simulink model "SoftStart"  (R2021a)
settings: Solver=ode45  StartTime=0.0  StopTime=10  RelTol=1e-3  EnableMultiTasking=on
undefined symbols (not defined in the file or in its folder): D1, lagging, pulse
libraries: spsThyristorLib x6, spsACVoltageSourceLib x3, spsAsynchronousMachineSIUnitsLib x2, spsThreePhaseVIMeasurementLib x2, spsPulseGeneratorThyristor12PulseLib x1, spsGroundLib x1, spsPLL3phLib x1, spspowerguiLib x1
settings Model: Creator=khaled18  LastModifiedBy=dudekpob
settings SolverCC: AlgebraicLoopSolver=TrustRegion
settings DataIOCC: LimitDataPoints=on  SaveFormat=Array  ReturnWorkspaceOutputs=off
settings OptimizationCC: LifeSpan=inf
settings DebuggingCC: SolverPrmCheckMsg=warning  SFUnexpectedBacktrackingDiag=warning  SFNoUnconditionalDefaultTransitionDiag=warning  SFExecutionAtInitializationDiag=none  SFMachineParentedDataDiag=warning  ArithmeticOperatorsInVariantConditions=warning
settings HardwareCC: ProdBitPerPointer=32  ProdBitPerSizeT=32  ProdBitPerPtrDiffT=32  ProdLargestAtomicFloat=None  ProdIntDivRoundTo=Undefined  ProdEndianess=Unspecified  ProdWordSize=32  ProdHWDeviceType=32-bit Generic
settings ModelReferenceCC: PropagateSignalLabelsOutOfModel=off
settings SFSimCC: SimUseLocalCustomCode=off  CustomCodeUndefinedFunction=UseInterfaceOnly
settings RTWCC: RTWUseLocalCustomCode=off
settings CodeAppCC: StateflowObjectComments=on
settings GRTTargetCC: TargetLangStandard=C89/C90 (ANSI)
settings ConfigComp: CovMetricSettings=dw  CovSaveCumulativeToWorkspaceVar=on  CovSaveSingleToWorkspaceVar=on  CovExternalEMLEnable=off  CovSFcnEnable=off
settings SimscapeCC: SimscapeNormalizeSystem=off

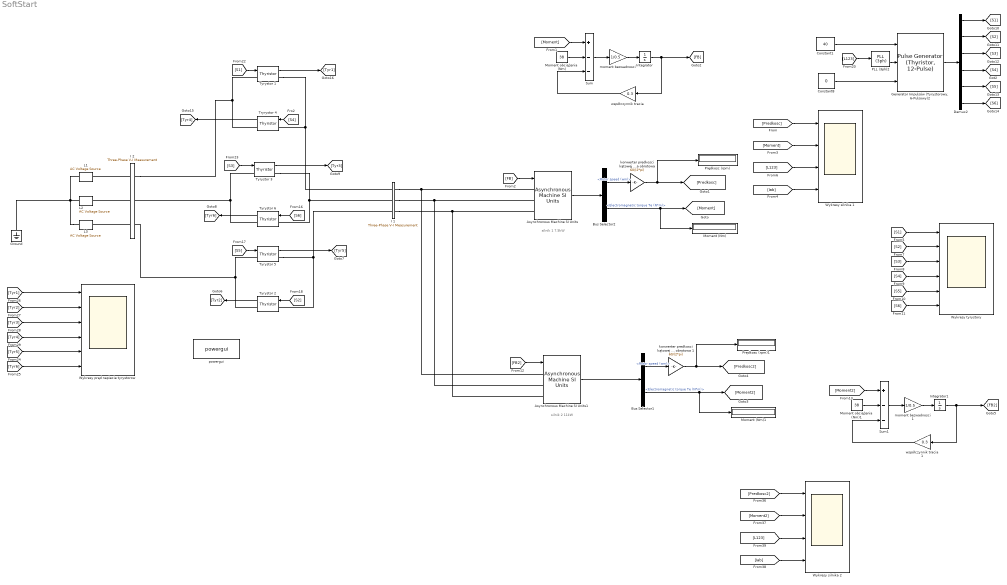
== system SoftStart ==
  note: silnik 1 7.5kW
  note: silnik 2 11kW
  Asynchronous Machine SI Units : spsAsynchronousMachineSIUnitsLib/Asynchronous Machine SI Units  RotorType=Squirrel-cage  PresetModel=No  MechanicalLoad=Speed w  ShowDetailedParameters=on  ReferenceFrame=Rotor  Units=SI  MeasurementBus=off  NominalParameters=[7500 400 50]  VoltageRatio=1  Stator=[1.405 0.005839]  Rotor=[1.395 0.005839]  Cage1=[ 0.022 0.226/377]  Cage2=[ 0.022 0.226/377]  Lm=0.1722  Mechanical=[0.0131 0.002985 3]  PolePairs=3  InitialConditions=[1 0 0 0 0 0 0 0]  SimulateSaturation=on  Saturation=[14.03593122, 27.81365428, 53.79336849, 72.68890987, 97.98006896, 148.6815601, 215.7428561, 302.9841135, 428.7778367 ; 230, 322, 414, 460, 506, 552, 598, 644, 690]  LoadFlowParameters=1492000  TsPowergui=0  TsBlock=-1  IterativeModel=Forward Euler  IterativeDiscreteModel=Trapezoidal non iterative  Pmec=0
      settings: AttributesFormatString=\n
  Asynchronous Machine SI Units1 : spsAsynchronousMachineSIUnitsLib/Asynchronous Machine SI Units  RotorType=Squirrel-cage  PresetModel=No  MechanicalLoad=Speed w  ShowDetailedParameters=on  ReferenceFrame=Rotor  Units=SI  MeasurementBus=off  NominalParameters=[11000 400 50]  VoltageRatio=1  Stator=[1.405 0.005839]  Rotor=[1.395 0.005839]  Cage1=[ 0.022 0.226/377]  Cage2=[ 0.022 0.226/377]  Lm=0.1722  Mechanical=[0.0131 0.002985 3]  PolePairs=3  InitialConditions=[1 0 0 0 0 0 0 0]  SimulateSaturation=on  Saturation=[14.03593122, 27.81365428, 53.79336849, 65.68890987, 75.98006896, 85.6815601, 90.7428561, 100.9841135, 110.7778367 ; 230, 322, 414, 460, 506, 552, 598, 644, 690]  LoadFlowParameters=1492000  TsPowergui=0  TsBlock=-1  IterativeModel=Forward Euler  IterativeDiscreteModel=Trapezoidal non iterative  Pmec=0
      settings: AttributesFormatString=\n
  Bus Selector1 : BusSelector  OutputSignals=Mechanical.Rotor speed (wm),Mechanical.Electromagnetic torque Te (N*m)
  Bus Selector2 : BusSelector  OutputSignals=Mechanical.Rotor speed (wm),Mechanical.Electromagnetic torque Te (N*m)
  Constant1 : Constant  Value=40
  Constant8 : Constant  Value=0
  Demux2 : Demux  Outputs=6
  "Generator Impulsów (Tyrystorowy, 6-Pulsowy)2" : spsPulseGeneratorThyristor12PulseLib/Pulse Generator (Thyristor, 12-Pulse)  GenType=6-pulse  Delta=D1 (lagging)  pwidth=50  Double_Pulse=on  Ts=0
      settings: SourceProductBaseCode=PS
  Ground : spsGroundLib/Ground  LConnTagsString=a
  I 1 : spsThreePhaseVIMeasurementLib/Three-Phase V-I Measurement  VoltageMeasurement=phase-to-phase  SetLabelV=on  LabelV=Vabc1  Vpu=off  VpuLL=off  CurrentMeasurement=yes  SetLabelI=on  LabelI=Iabc1  Ipu=off  Pbase=100e6  Vbase=500e3  OutputType=Complex  PhasorSimulation=off  PSBequivalent=0
  I 2 : spsThreePhaseVIMeasurementLib/Three-Phase V-I Measurement  VoltageMeasurement=phase-to-ground  SetLabelV=on  LabelV=L123  Vpu=off  VpuLL=off  CurrentMeasurement=yes  SetLabelI=on  LabelI=Iab  Ipu=off  Pbase=100e6  Vbase=500e3  OutputType=Complex  PhasorSimulation=off  PSBequivalent=0
  Integrator : Integrator
  Integrator1 : Integrator
  L1 : spsACVoltageSourceLib/AC Voltage Source  Amplitude=400  Phase=0  Frequency=50  SampleTime=0  Measurements=None  BusType=swing  Pref=10e3  Qref=0  Qmin=-inf  Qmax=+inf
  L2 : spsACVoltageSourceLib/AC Voltage Source  Amplitude=400  Phase=-120  Frequency=50  SampleTime=0  Measurements=None  BusType=swing  Pref=10e3  Qref=0  Qmin=-inf  Qmax=+inf
  L3 : spsACVoltageSourceLib/AC Voltage Source  Amplitude=400  Phase=120  Frequency=50  SampleTime=0  Measurements=None  BusType=swing  Pref=10e3  Qref=0  Qmin=-inf  Qmax=+inf
  Moment (Nm) : Display
  Moment (Nm)1 : Display
  Moment obciążenia  (Nm) : Constant  Value=38
  Moment obciążenia  (Nm)1 : Constant  Value=38
  PLL (3ph)2 : spsPLL3phLib/PLL (3ph)  Fmin=45  Par_Init=[0, 50]  ParK=[180, 3200, 1]  TcD=1e-4  MaxRateChangeFreq=12  FilterCutOffFreq=25  Ts=0  AGC=on
  Prędkosc (rpm) : Display
  Prędkosc (rpm)1 : Display
  Sum : Sum  Inputs=+--
  Sum1 : Sum  Inputs=+--
  Tryrystor 4 : spsThyristorLib/Thyristor  Ron=0.001  Lon=0  Vf=0.8  IC=0  Rs=500  Cs=250e-9  Measurements=on
  Tyrystor {1..3,5..6} (5 alike) : spsThyristorLib/Thyristor  Ron=0.001  Lon=0  Vf=0.8  IC=0  Rs=500  Cs=250e-9  Measurements=on
  Wykresy prąd napiecie tyrystorow : Scope  NumInputPorts=6
  Wykresy silnika 1 : Scope  NumInputPorts=4
  Wykresy silnika 2 : Scope  NumInputPorts=4
  Wykresy tyrystory : Scope  NumInputPorts=6
  "konwerter predkosci kątowej na obrotowa " : Gain  Gain=60/(2*pi)
  konwerter predkosci kątowej na obrotowa 1 : Gain  Gain=60/(2*pi)
  moment bezwadnosci : Gain  Gain=1/0.5
  moment bezwadnosci1 : Gain  Gain=1/0.5
  powergui : spspowerguiLib/powergui  Priority=1  SimulationMode=Discrete  SampleTime=50e-6  frequency=60  Iterations=50  frequencyindice=50  Pbase=100e6  ErrMax=1e-4  UnitsV=kV  UnitsW=MW  buscounter=0  FunctionMessages=off  echomessages=off  EnableUseOfTLC=off  CurrentSourceSwitches=off  DisableSnubberDevices=off  DisableRonSwitches=off  DisableVfSwitches=off  DisplayEquations=off  AutomaticDiscreteSolvers=off  SolverType=Tustin/Backward Euler (TBE)  Interpol=off  ExternalGateDelay=off  methode=off  Ts=100  x0status=blocks  SPID=off  SwTol=0  HookPort=off  NonlinearTolerance=1e-4  nMaxIteration=100  ContinueOnMaxIteration=off  RestoreLinks=warning  ResistiveCurrentMeasurement=off  Frange=[0:2:500]  Ylog=off  Xlog=on  ShowGrid=off  save=off  variable=ZData  structure=0  ZoomFFT=off  StartTime=0.0  cycles=1  DisplayStyle=1  fundamental=60  FreqAxis=off  MaxFrequency=1000  frequencyindicesteady=1  RmsSteady=1  display=off
  "współczynnik tracia " : Gain  Gain=0.3
  współczynnik tracia 1 : Gain  Gain=0.3
  wires:
  [L123] -> PLL (3ph)2/1
  Constant8/1 -> "Generator Impulsów (Tyrystorowy, 6-Pulsowy)2"/3
  "Generator Impulsów (Tyrystorowy, 6-Pulsowy)2"/1 -> Demux2/1
  [S4] -> Tryrystor 4/1
  [S5] -> Tyrystor 5/1
  Demux2/4 -> [S4]
  Asynchronous Machine SI Units/1 -> Bus Selector2/1
  [S6] -> Tyrystor 6/1
  Demux2/5 -> [S5]
  Demux2/2 -> [S2]
  Demux2/6 -> [S6]
  PLL (3ph)2/2 -> "Generator Impulsów (Tyrystorowy, 6-Pulsowy)2"/2
  [S1] -> Tyrystor 1/1
  Demux2/1 -> [S1]
  [S3] -> Tyrystor 3/1
  Demux2/3 -> [S3]
  [S2] -> Tyrystor 2/1
  Constant1/1 -> "Generator Impulsów (Tyrystorowy, 6-Pulsowy)2"/1
  Bus Selector2/2 -> Moment (Nm)/1, [Moment]  "<Electromagnetic torque Te (N*m)>"
  Sum/1 -> moment bezwadnosci/1
  moment bezwadnosci/1 -> Integrator/1
  Integrator/1 -> "współczynnik tracia "/1, [FB]
  Bus Selector2/1 -> "konwerter predkosci kątowej na obrotowa "/1  "<Rotor speed (wm)>"
  [Moment] -> Sum/1
  Moment obciążenia  (Nm)/1 -> Sum/2
  "współczynnik tracia "/1 -> Sum/3
  [FB] -> Asynchronous Machine SI Units/1
  "konwerter predkosci kątowej na obrotowa "/1 -> Prędkosc (rpm)/1, [Predkosc]
  [Predkosc] -> Wykresy silnika 1/1
  [Moment] -> Wykresy silnika 1/2
  [L123] -> Wykresy silnika 1/3
  [Iab] -> Wykresy silnika 1/4
  [S1] -> Wykresy tyrystory/1
  [S2] -> Wykresy tyrystory/2
  [S3] -> Wykresy tyrystory/3
  [S4] -> Wykresy tyrystory/4
  [S5] -> Wykresy tyrystory/5
  [S6] -> Wykresy tyrystory/6
  [Tyr4] -> Wykresy prąd napiecie tyrystorow/4
  [Tyr1] -> Wykresy prąd napiecie tyrystorow/1
  [Tyr3] -> Wykresy prąd napiecie tyrystorow/3
  [Tyr2] -> Wykresy prąd napiecie tyrystorow/2
  [Tyr6] -> Wykresy prąd napiecie tyrystorow/6
  [Tyr5] -> Wykresy prąd napiecie tyrystorow/5
  Tyrystor 2/1 -> [Tyr2]
  Tyrystor 5/1 -> [Tyr5]
  Tyrystor 6/1 -> [Tyr6]
  Tyrystor 3/1 -> [Tyr3]
  Tryrystor 4/1 -> [Tyr4]
  Tyrystor 1/1 -> [Tyr1]
  [Predkosc2] -> Wykresy silnika 2/1
  [Iab] -> Wykresy silnika 2/4
  [Moment2] -> Wykresy silnika 2/2
  [L123] -> Wykresy silnika 2/3
  [FB2] -> Asynchronous Machine SI Units1/1
  Bus Selector1/1 -> konwerter predkosci kątowej na obrotowa 1/1  "<Rotor speed (wm)>"
  konwerter predkosci kątowej na obrotowa 1/1 -> Prędkosc (rpm)1/1, [Predkosc2]
  Bus Selector1/2 -> Moment (Nm)1/1, [Moment2]  "<Electromagnetic torque Te (N*m)>"
  moment bezwadnosci1/1 -> Integrator1/1
  [Moment2] -> Sum1/1
  Moment obciążenia  (Nm)1/1 -> Sum1/2
  współczynnik tracia 1/1 -> Sum1/3
  Integrator1/1 -> współczynnik tracia 1/1, [FB2]
  Asynchronous Machine SI Units1/1 -> Bus Selector1/1
  Sum1/1 -> moment bezwadnosci1/1
  connections:
  I 2/RConn1 -- Tryrystor 4/RConn1 -- Tyrystor 1/LConn1
  Tyrystor 5/LConn1 -- Tyrystor 2/RConn1 -- I 2/RConn3
  Tyrystor 3/LConn1 -- Tyrystor 6/RConn1 -- I 2/RConn2
  I 1/LConn2 -- Tyrystor 3/RConn1 -- Tyrystor 6/LConn1
  L3/LConn1 -- Ground/LConn1 -- L2/LConn1 -- L1/LConn1
  I 1/LConn3 -- Tyrystor 5/RConn1 -- Tyrystor 2/LConn1
  I 1/LConn1 -- Tyrystor 1/RConn1 -- Tryrystor 4/LConn1
  I 2/LConn3 -- L3/RConn1
  I 2/LConn2 -- L2/RConn1
  I 2/LConn1 -- L1/RConn1
  I 1/RConn1 -- Asynchronous Machine SI Units1/LConn1 -- Asynchronous Machine SI Units/LConn1
  I 1/RConn2 -- Asynchronous Machine SI Units1/LConn2 -- Asynchronous Machine SI Units/LConn2
  I 1/RConn3 -- Asynchronous Machine SI Units1/LConn3 -- Asynchronous Machine SI Units/LConn3
